simulink model "compare_f_w"  (R2015b)
settings: Solver=VariableStepAuto  StartTime=0.0  StopTime=10  RelTol=1e-3
libraries: dspsrcs4 x1
settings Model: Creator=YogurtSuee  LastModifiedBy=YogurtSuee

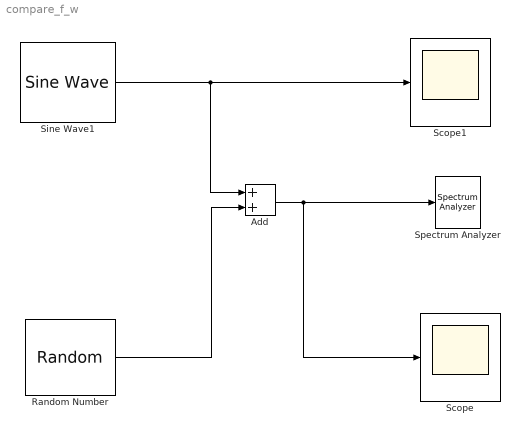
== system compare_f_w ==
  Add : Sum
  Random Number : RandomNumber  Variance=0.1  SampleTime=0.01
  Scope : Scope
  Scope1 : Scope
  Sine Wave1 : dspsrcs4/Sine Wave  Amplitude=5  Frequency=50  Phase=0  SampleMode=Discrete  OutComplex=Real  CompMethod=Trigonometric fcn  TableSize=Speed  SampleTime=1/1000  SamplesPerFrame=1  ResetState=Restart at time zero  OutputFrames=off  dataType=double  wordLen=16  udDataType=sfix(16)  fracBitsMode=Best precision  numFracBits=15  OutDataTypeStr=double  LastOutDataTypeStr=double
  Spectrum Analyzer : SpectrumAnalyzer
  wires:
  Add/1 -> Scope/1, Spectrum Analyzer/1
  Sine Wave1/1 -> Add/1, Scope1/1
  Random Number/1 -> Add/2
